simulink model "c00016"  (R2018a)
settings: Solver=FixedStepAuto  StartTime=0.0  StopTime=300  FixedStep=0.1  RelTol=1e-3
undefined symbols (not defined in the file): A1, hmax, PriorityTank, R1, R2
settings Model: Creator=aarrieta  LastModifiedBy=umarkiegi

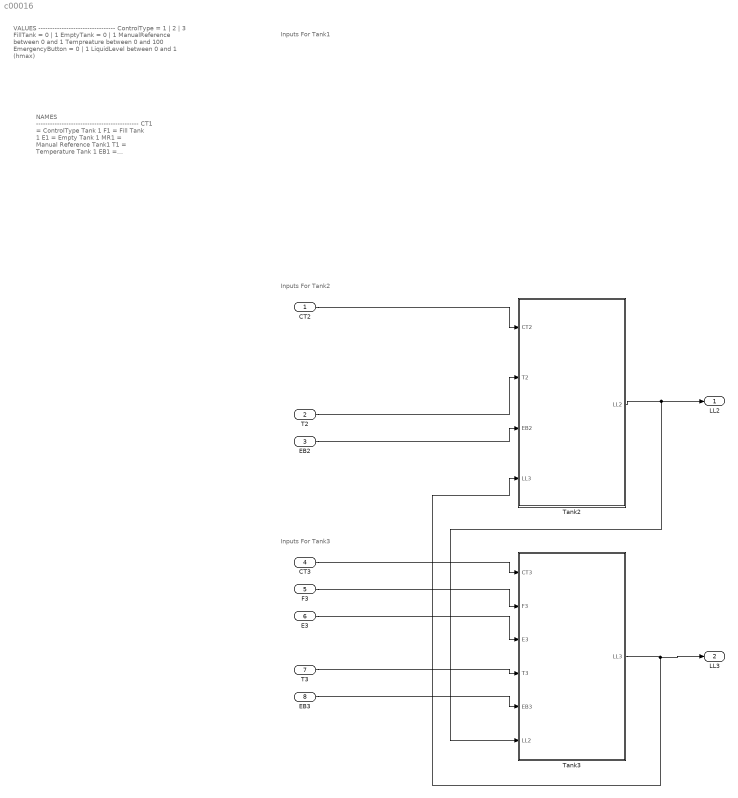
== system c00016 ==
  note: Inputs For Tank1
  note: VALUES
      | ---------------------------------
      | ControlType = 1 | 2 | 3
      | FillTank = 0 | 1
      | EmptyTank = 0 | 1
      | ManualReference between 0 and 1
      | Tempreature between 0 and 100
      | EmergencyButton = 0 | 1
      | LiquidLevel between 0 and 1 (hmax)
  note: NAMES
      | --------------------------------------------
      | CT1 = ControlType Tank 1
      | F1 = Fill Tank 1
      | E1 = Empty Tank 1
      | MR1 = Manual Reference Tank1
      | T1 = Temperature Tank 1
      | EB1 = Emergency Button Tank 1
      | LL1 = Liquid Level 1
  note: Inputs For Tank2
  note: Inputs For Tank3
  CT2 : Inport
  T2 : Inport  Port=2
  EB2 : Inport  Port=3
  CT3 : Inport  Port=4
  F3 : Inport  Port=5
  E3 : Inport  Port=6
  T3 : Inport  Port=7
  EB3 : Inport  Port=8
  Tank2 : Subsystem
  Tank3 : Subsystem
  LL2 : Outport
  LL3 : Outport  Port=2
  wires:
  Tank2/1(LL2) -> LL2/1, Tank3/6(LL2)
  Tank3/1(LL3) -> LL3/1, Tank2/4(LL3)
  CT2/1 -> Tank2/1(CT2)
  EB2/1 -> Tank2/3(EB2)
  T2/1 -> Tank2/2(T2)
  T3/1 -> Tank3/4(T3)
  EB3/1 -> Tank3/5(EB3)
  E3/1 -> Tank3/3(E3)
  F3/1 -> Tank3/2(F3)
  CT3/1 -> Tank3/1(CT3)

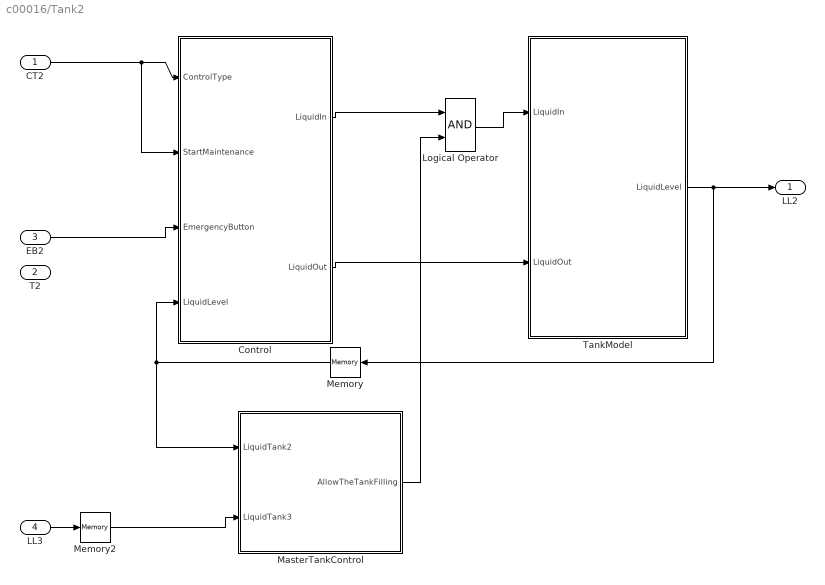
== system c00016/Tank2 ==
  CT2 : Inport
  T2 : Inport  Port=2
  EB2 : Inport  Port=3
  LL3 : Inport  Port=4
  Control : Subsystem
  Logical Operator : Logic  AllPortsSameDT=off  OutDataTypeStr=boolean
  MasterTankControl : Subsystem
  Memory : Memory
  Memory2 : Memory
  TankModel : Subsystem
  LL2 : Outport
  wires:
  TankModel/1(LiquidLevel) -> Memory/1, LL2/1
  Control/1(LiquidIn) -> Logical Operator/1
  Control/2(LiquidOut) -> TankModel/2(LiquidOut)
  Memory/1 -> Control/4(LiquidLevel), MasterTankControl/1(LiquidTank2)
  CT2/1 -> Control/2(StartMaintenance), Control/1(ControlType)
  LL3/1 -> Memory2/1
  Memory2/1 -> MasterTankControl/2(LiquidTank3)
  EB2/1 -> Control/3(EmergencyButton)
  MasterTankControl/1(AllowTheTankFilling) -> Logical Operator/2
  Logical Operator/1 -> TankModel/1(LiquidIn)

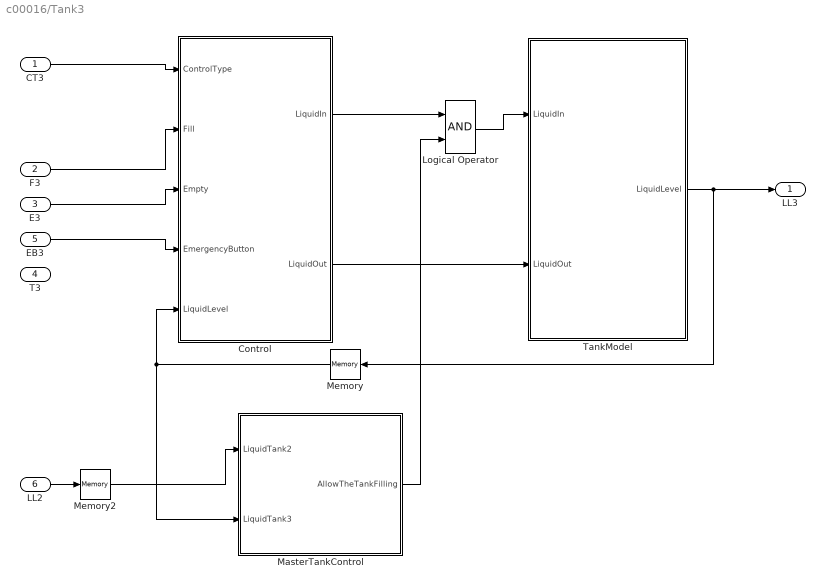
== system c00016/Tank3 ==
  CT3 : Inport
  F3 : Inport  Port=2
  E3 : Inport  Port=3
  T3 : Inport  Port=4
  EB3 : Inport  Port=5
  LL2 : Inport  Port=6
  Control : Subsystem
  Logical Operator : Logic  AllPortsSameDT=off  OutDataTypeStr=boolean
  MasterTankControl : Subsystem
  Memory : Memory
  Memory2 : Memory
  TankModel : Subsystem
  LL3 : Outport
  wires:
  TankModel/1(LiquidLevel) -> Memory/1, LL3/1
  Control/1(LiquidIn) -> Logical Operator/1
  Control/2(LiquidOut) -> TankModel/2(LiquidOut)
  Memory/1 -> MasterTankControl/2(LiquidTank3), Control/5(LiquidLevel)
  CT3/1 -> Control/1(ControlType)
  F3/1 -> Control/2(Fill)
  E3/1 -> Control/3(Empty)
  LL2/1 -> Memory2/1
  Memory2/1 -> MasterTankControl/1(LiquidTank2)
  EB3/1 -> Control/4(EmergencyButton)
  MasterTankControl/1(AllowTheTankFilling) -> Logical Operator/2
  Logical Operator/1 -> TankModel/1(LiquidIn)

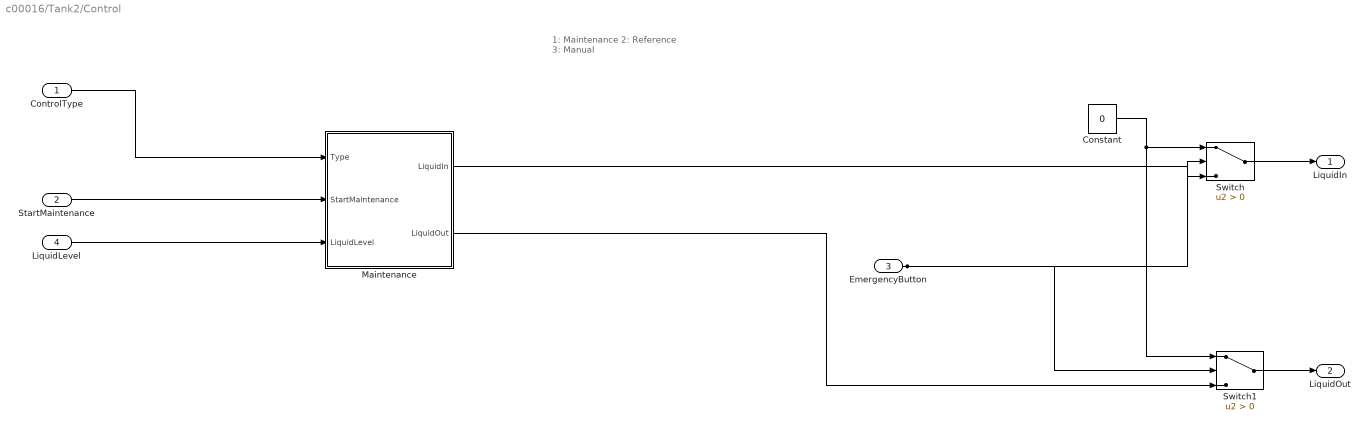
== system c00016/Tank2/Control ==
  note: 1: Maintenance
      | 2: Reference
      | 3: Manual
  ControlType : Inport
  StartMaintenance : Inport  Port=2
  EmergencyButton : Inport  Port=3
  LiquidLevel : Inport  Port=4
  Constant : Constant  Value=0
  Maintenance : Subsystem
  Switch : Switch  Criteria=u2 > Threshold
  Switch1 : Switch  Criteria=u2 > Threshold
  LiquidIn : Outport
  LiquidOut : Outport  Port=2
  wires:
  ControlType/1 -> Maintenance/1(Type)
  LiquidLevel/1 -> Maintenance/3(LiquidLevel)
  StartMaintenance/1 -> Maintenance/2(StartMaintenance)
  Switch/1 -> LiquidIn/1
  Switch1/1 -> LiquidOut/1
  Constant/1 -> Switch1/1, Switch/1
  EmergencyButton/1 -> Switch/2, Switch1/2
  Maintenance/1(LiquidIn) -> Switch/3
  Maintenance/2(LiquidOut) -> Switch1/3

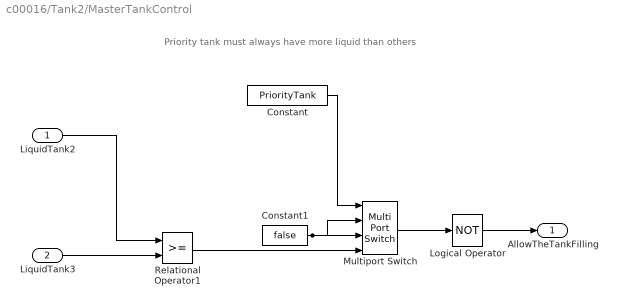
== system c00016/Tank2/MasterTankControl ==
  note: Priority tank must always have more liquid than others
  LiquidTank2 : Inport
  LiquidTank3 : Inport  Port=2
  Constant : Constant  Value=PriorityTank
  Constant1 : Constant  Value=false
  Logical Operator : Logic  Operator=NOT  AllPortsSameDT=off  OutDataTypeStr=boolean
  Multiport Switch : MultiPortSwitch
  Relational Operator1 : RelationalOperator  OutDataTypeStr=boolean  RndMeth=Simplest
  AllowTheTankFilling : Outport
  wires:
  LiquidTank2/1 -> Relational Operator1/1
  LiquidTank3/1 -> Relational Operator1/2
  Constant/1 -> Multiport Switch/1
  Relational Operator1/1 -> Multiport Switch/4
  Constant1/1 -> Multiport Switch/3, Multiport Switch/2
  Multiport Switch/1 -> Logical Operator/1
  Logical Operator/1 -> AllowTheTankFilling/1

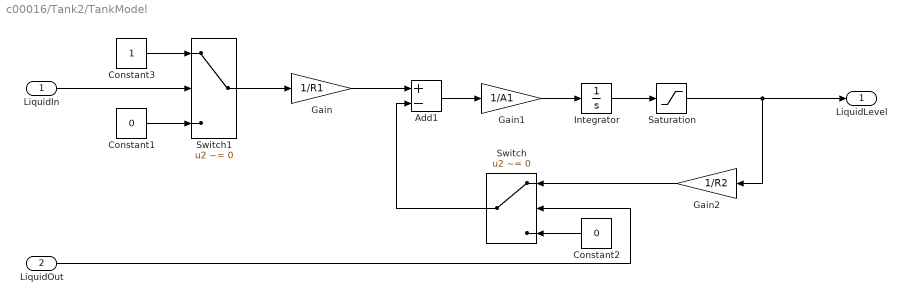
== system c00016/Tank2/TankModel ==
  LiquidIn : Inport
  LiquidOut : Inport  Port=2
  Add1 : Sum  Inputs=+-
  Constant1 : Constant  Value=0
  Constant2 : Constant  Value=0
  Constant3 : Constant
  Gain : Gain  Gain=1/R1
  Gain1 : Gain  Gain=1/A1
  Gain2 : Gain  Gain=1/R2
  Integrator : Integrator
  Saturation : Saturate  UpperLimit=hmax  LowerLimit=0
  Switch : Switch  Criteria=u2 ~= 0
  Switch1 : Switch  Criteria=u2 ~= 0
  LiquidLevel : Outport
  wires:
  Saturation/1 -> LiquidLevel/1, Gain2/1
  LiquidOut/1 -> Switch/2
  Add1/1 -> Gain1/1
  Gain2/1 -> Switch/1
  LiquidIn/1 -> Switch1/2
  Switch/1 -> Add1/2
  Switch1/1 -> Gain/1
  Constant2/1 -> Switch/3
  Constant3/1 -> Switch1/1
  Integrator/1 -> Saturation/1
  Gain1/1 -> Integrator/1
  Gain/1 -> Add1/1
  Constant1/1 -> Switch1/3

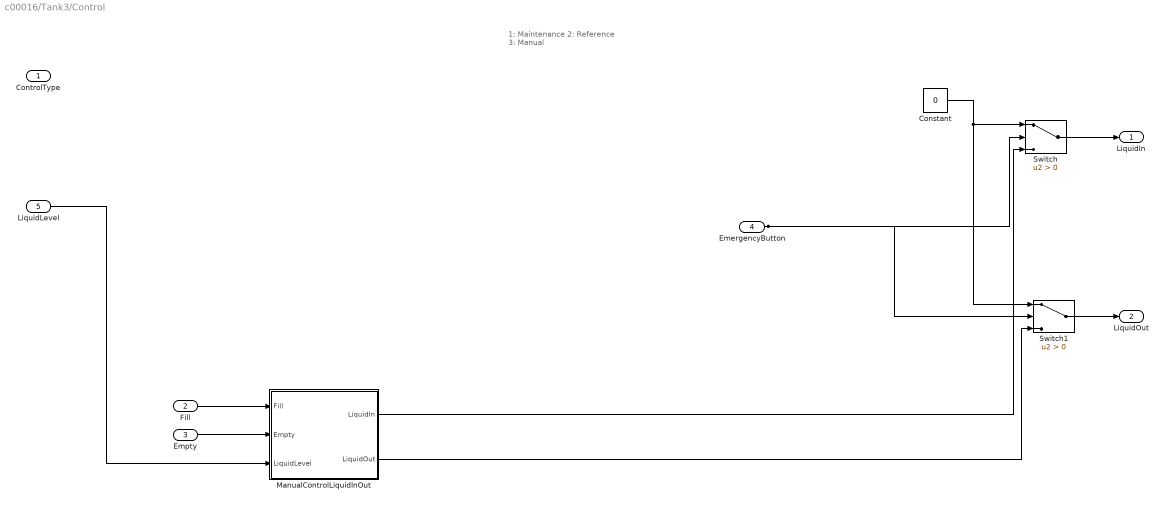
== system c00016/Tank3/Control ==
  note: 1: Maintenance
      | 2: Reference
      | 3: Manual
  ControlType : Inport
  Fill : Inport  Port=2
  Empty : Inport  Port=3
  EmergencyButton : Inport  Port=4
  LiquidLevel : Inport  Port=5
  Constant : Constant  Value=0
  ManualControlLiquidInOut : Subsystem
  Switch : Switch  Criteria=u2 > Threshold
  Switch1 : Switch  Criteria=u2 > Threshold
  LiquidIn : Outport
  LiquidOut : Outport  Port=2
  wires:
  LiquidLevel/1 -> ManualControlLiquidInOut/3(LiquidLevel)
  Empty/1 -> ManualControlLiquidInOut/2(Empty)
  Fill/1 -> ManualControlLiquidInOut/1(Fill)
  Switch/1 -> LiquidIn/1
  Switch1/1 -> LiquidOut/1
  Constant/1 -> Switch1/1, Switch/1
  EmergencyButton/1 -> Switch/2, Switch1/2
  ManualControlLiquidInOut/1(LiquidIn) -> Switch/3
  ManualControlLiquidInOut/2(LiquidOut) -> Switch1/3

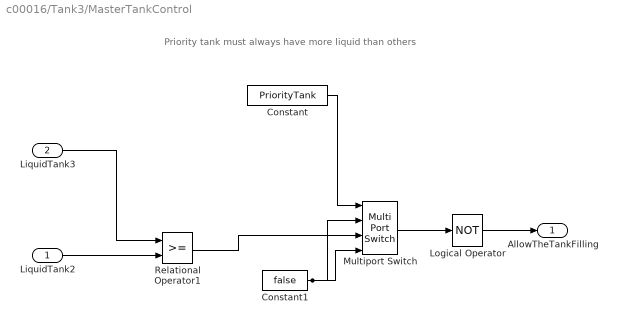
== system c00016/Tank3/MasterTankControl ==
  note: Priority tank must always have more liquid than others
  LiquidTank2 : Inport
  LiquidTank3 : Inport  Port=2
  Constant : Constant  Value=PriorityTank
  Constant1 : Constant  Value=false
  Logical Operator : Logic  Operator=NOT  AllPortsSameDT=off  OutDataTypeStr=boolean
  Multiport Switch : MultiPortSwitch
  Relational Operator1 : RelationalOperator  OutDataTypeStr=boolean  RndMeth=Simplest
  AllowTheTankFilling : Outport
  wires:
  Constant/1 -> Multiport Switch/1
  Relational Operator1/1 -> Multiport Switch/3
  Constant1/1 -> Multiport Switch/4, Multiport Switch/2
  Multiport Switch/1 -> Logical Operator/1
  Logical Operator/1 -> AllowTheTankFilling/1
  LiquidTank2/1 -> Relational Operator1/2
  LiquidTank3/1 -> Relational Operator1/1

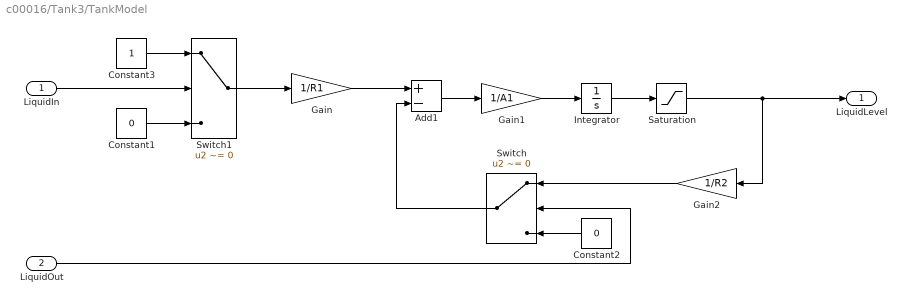
== system c00016/Tank3/TankModel ==
  LiquidIn : Inport
  LiquidOut : Inport  Port=2
  Add1 : Sum  Inputs=+-
  Constant1 : Constant  Value=0
  Constant2 : Constant  Value=0
  Constant3 : Constant
  Gain : Gain  Gain=1/R1
  Gain1 : Gain  Gain=1/A1
  Gain2 : Gain  Gain=1/R2
  Integrator : Integrator
  Saturation : Saturate  UpperLimit=hmax  LowerLimit=0
  Switch : Switch  Criteria=u2 ~= 0
  Switch1 : Switch  Criteria=u2 ~= 0
  LiquidLevel : Outport
  wires:
  Saturation/1 -> LiquidLevel/1, Gain2/1
  LiquidOut/1 -> Switch/2
  Add1/1 -> Gain1/1
  Gain2/1 -> Switch/1
  LiquidIn/1 -> Switch1/2
  Switch/1 -> Add1/2
  Switch1/1 -> Gain/1
  Constant2/1 -> Switch/3
  Constant3/1 -> Switch1/1
  Integrator/1 -> Saturation/1
  Gain1/1 -> Integrator/1
  Gain/1 -> Add1/1
  Constant1/1 -> Switch1/3

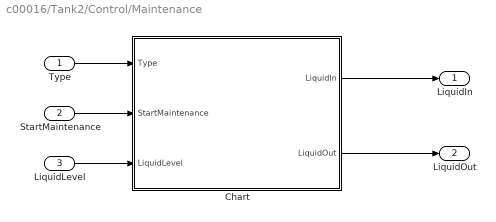
== system c00016/Tank2/Control/Maintenance ==
  Type : Inport
  StartMaintenance : Inport  Port=2
  LiquidLevel : Inport  Port=3
  Chart : Stateflow chart  TreatAsAtomicUnit=on
  LiquidIn : Outport
  LiquidOut : Outport  Port=2
  wires:
  StartMaintenance/1 -> Chart/2(StartMaintenance)
  Type/1 -> Chart/1(Type)
  LiquidLevel/1 -> Chart/3(LiquidLevel)
  Chart/1(LiquidIn) -> LiquidIn/1
  Chart/2(LiquidOut) -> LiquidOut/1

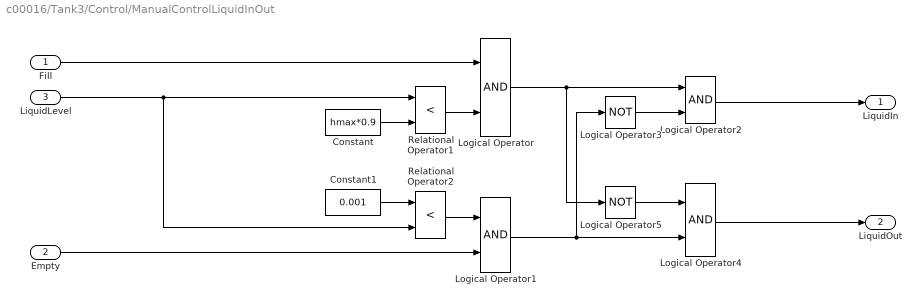
== system c00016/Tank3/Control/ManualControlLiquidInOut ==
  Fill : Inport
  Empty : Inport  Port=2
  LiquidLevel : Inport  Port=3
  Constant : Constant  Value=hmax*0.9
  Constant1 : Constant  Value=0.001
  Logical Operator{,1..2,4} (4 alike) : Logic  AllPortsSameDT=off  OutDataTypeStr=boolean
  Logical Operator3 : Logic  Operator=NOT  AllPortsSameDT=off  OutDataTypeStr=boolean
  Logical Operator5 : Logic  Operator=NOT  AllPortsSameDT=off  OutDataTypeStr=boolean
  Relational Operator1 : RelationalOperator  Operator=<  OutDataTypeStr=boolean  RndMeth=Simplest
  Relational Operator2 : RelationalOperator  Operator=<  OutDataTypeStr=boolean  RndMeth=Simplest
  LiquidIn : Outport
  LiquidOut : Outport  Port=2
  wires:
  Empty/1 -> Logical Operator1/2
  Constant/1 -> Relational Operator1/2
  Relational Operator1/1 -> Logical Operator/2
  Fill/1 -> Logical Operator/1
  Logical Operator/1 -> Logical Operator5/1, Logical Operator2/1
  Relational Operator2/1 -> Logical Operator1/1
  Logical Operator1/1 -> Logical Operator3/1, Logical Operator4/2
  Constant1/1 -> Relational Operator2/1
  LiquidLevel/1 -> Relational Operator2/2, Relational Operator1/1
  Logical Operator3/1 -> Logical Operator2/2
  Logical Operator2/1 -> LiquidIn/1
  Logical Operator5/1 -> Logical Operator4/1
  Logical Operator4/1 -> LiquidOut/1

== stateflow chart c00016/Tank2/Control/Maintenance/Chart ==
  state InitialState
    entry: LiquidIn = 0;
    LiquidOut = 0;
  state Step1
    entry: LiquidIn = 0;
    LiquidOut = 1;
  state Step2
    entry: LiquidIn = 1;
    LiquidOut = 0;
  state Step3
    entry: LiquidIn = 0;
    LiquidOut = 1;
  (default) -> InitialState
  Step3 -> InitialState : [Type~=1||LiquidLevel <=0.01]
  Step2 -> InitialState [order 1] : [Type~=1]
  Step1 -> InitialState [order 1] : [Type ~= 1]
  InitialState -> Step1 : [StartMaintenance == 1 && Type ==1]
  Step1 -> Step2 [order 2] : [LiquidLevel <=0.01]
  Step2 -> Step3 [order 2] : [LiquidLevel>=hmax*0.9]
  data: Type input; StartMaintenance input; LiquidIn output; LiquidOut output; LiquidLevel input; hmax parameter
